simulink model "ACMtr_demo"  (R2019b)
settings: Solver=VariableStepAuto  StartTime=0.0  StopTime=2  RelTol=1e-3
libraries: powerlib x12, simulink x1
settings Model: Creator=DELL  LastModifiedBy=DELL

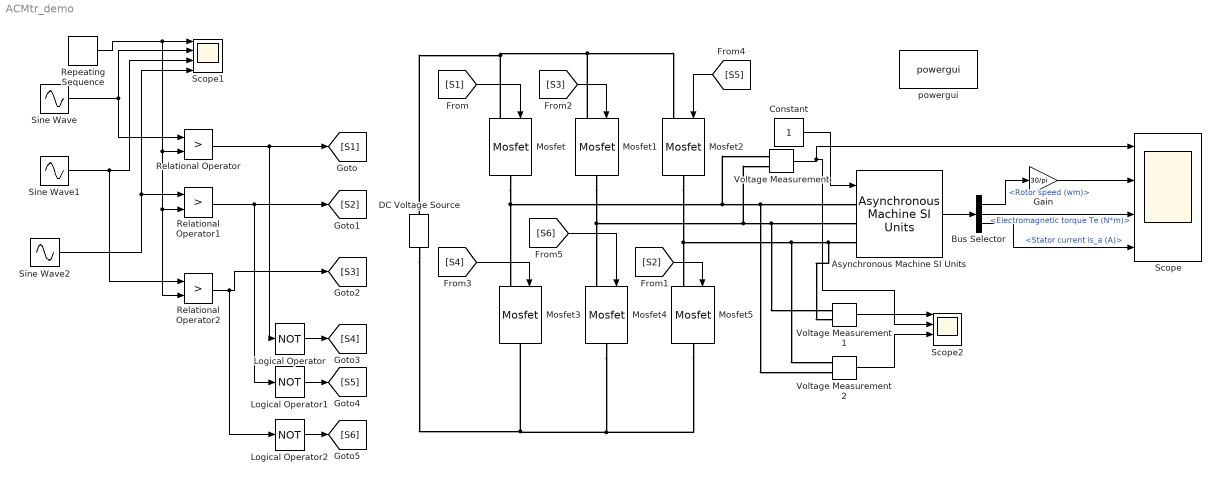
== system ACMtr_demo ==
  Asynchronous Machine SI Units : powerlib/Machines/Asynchronous Machine SI Units  RotorType=Squirrel-cage  PresetModel="15:  5.4 HP (4KW)   400 V  50Hz 1430 RPM"  MechanicalLoad=Torque Tm  ShowDetailedParameters=on  ReferenceFrame=Rotor  Units=SI  MeasurementBus=off  NominalParameters=[4000 400 50]  Stator=[1.405 0.005839]  Rotor=[1.395 0.005839]  Cage1=[0.4155 0.002066]  Cage2=[0.4168 0.0003495]  Lm=0.1722  Mechanical=[0.0131 0.002985 2]  PolePairs=2  InitialConditions=[0 0 0 0 0 0 0 0]  SimulateSaturation=off  Saturation=[14.03593122, 27.81365428, 53.79336849, 72.68890987, 97.98006896, 148.6815601, 215.7428561, 302.9841135, 428.7778367 ; 230, 322, 414, 460, 506, 552, 598, 644, 690]  LoadFlowParameters=1492000  TsPowergui=0  TsBlock=-1  IterativeModel=Trapezoidal non iterative  IterativeDiscreteModel=Trapezoidal non iterative  Pmec=1.492e+006
      settings: SourceProductName=Simscape Electrical
  Bus Selector : BusSelector  OutputSignals=Mechanical.Rotor speed (wm),Mechanical.Electromagnetic torque Te (N*m),Stator measurements.Stator current is_a (A)
  Constant : Constant
  DC Voltage Source : powerlib/Electrical Sources/DC Voltage Source  Amplitude=600  Measurements=None
      settings: SourceProductName=Simscape Electrical
  Gain : Gain  Gain=30/pi
  Logical Operator : Logic  Operator=NOT  AllPortsSameDT=off  OutDataTypeStr=boolean
  Logical Operator1 : Logic  Operator=NOT  AllPortsSameDT=off  OutDataTypeStr=boolean
  Logical Operator2 : Logic  Operator=NOT  AllPortsSameDT=off  OutDataTypeStr=boolean
  Mosfet{,1..5} (6 alike) : powerlib/Power Electronics/Mosfet  Ron=0.1  Lon=0  Rd=0.01  Vfd=0  IC=0  Rs=1e5  Cs=inf  Measurements=off
      settings: SourceProductName=Simscape Electrical
  Relational Operator : RelationalOperator  Operator=>  OutDataTypeStr=boolean  RndMeth=Simplest
  Relational Operator1 : RelationalOperator  Operator=>  OutDataTypeStr=boolean  RndMeth=Simplest
  Relational Operator2 : RelationalOperator  Operator=>  OutDataTypeStr=boolean  RndMeth=Simplest
  Repeating Sequence : simulink/Sources/Repeating Sequence  rep_seq_t=[0 0.25 0.5 0.75 1]/5000  rep_seq_y=[0 1 0 -1 0]
  Scope : Scope  NumInputPorts=4
  Scope1 : Scope  NumInputPorts=4
  Scope2 : Scope  NumInputPorts=4
  Sine Wave : Sin  Amplitude=0.6  Frequency=2*pi*50  SampleTime=0
  Sine Wave1 : Sin  Amplitude=0.6  Frequency=2*pi*50  Phase=120*pi/180  SampleTime=0
  Sine Wave2 : Sin  Amplitude=0.6  Frequency=2*pi*50  Phase=240*pi/180  SampleTime=0
  Voltage Measurement : powerlib/Measurements/Voltage Measurement  PhasorSimulation=off  OutputType=Complex  PSBequivalent=0
      settings: SourceProductName=Simscape Electrical
  Voltage Measurement1 : powerlib/Measurements/Voltage Measurement  PhasorSimulation=off  OutputType=Complex  PSBequivalent=0
      settings: SourceProductName=Simscape Electrical
  Voltage Measurement2 : powerlib/Measurements/Voltage Measurement  PhasorSimulation=off  OutputType=Complex  PSBequivalent=0
      settings: SourceProductName=Simscape Electrical
  powergui : powerlib/powergui  Priority=1  SimulationMode=Discrete  SampleTime=50e-6  frequency=60  Iterations=50  frequencyindice=50  Pbase=100e6  ErrMax=1e-4  UnitsV=kV  UnitsW=MW  buscounter=0  FunctionMessages=off  echomessages=off  EnableUseOfTLC=off  CurrentSourceSwitches=off  DisableSnubberDevices=off  DisableRonSwitches=off  DisableVfSwitches=off  DisplayEquations=off  AutomaticDiscreteSolvers=off  SolverType=Tustin/Backward Euler (TBE)  Interpol=off  ExternalGateDelay=off  methode=off  Ts=100  x0status=blocks  SPID=on  SwTol=0  HookPort=off  NonlinearTolerance=1e-4  nMaxIteration=100  ContinueOnMaxIteration=off  RestoreLinks=warning  ResistiveCurrentMeasurement=off  Frange=[0:2:500]  Ylog=off  Xlog=on  ShowGrid=off  save=off  variable=ZData  structure=0  ZoomFFT=off  StartTime=0.0  cycles=1  DisplayStyle=1  fundamental=60  FreqAxis=off  MaxFrequency=1000  frequencyindicesteady=1  RmsSteady=1  display=off
      settings: SourceProductName=Simscape Electrical
  wires:
  Relational Operator/1 -> Logical Operator/1, [S1]
  [S1] -> Mosfet/1
  [S2] -> Mosfet5/1
  Relational Operator2/1 -> Logical Operator2/1, [S3]
  [S3] -> Mosfet1/1
  Logical Operator/1 -> [S4]
  [S4] -> Mosfet3/1
  Logical Operator1/1 -> [S5]
  [S5] -> Mosfet2/1
  Logical Operator2/1 -> [S6]
  [S6] -> Mosfet4/1
  Constant/1 -> Asynchronous Machine SI Units/1
  Asynchronous Machine SI Units/1 -> Bus Selector/1
  Voltage Measurement/1 -> Scope2/2, Scope/1
  Bus Selector/1 -> Gain/1  "<Rotor speed (wm)>"
  Bus Selector/2 -> Scope/3  "<Electromagnetic torque Te (N*m)>"
  Bus Selector/3 -> Scope/4  "<Stator current is_a (A)>"
  Gain/1 -> Scope/2
  Repeating Sequence/1 -> Relational Operator2/2, Relational Operator1/2, Relational Operator/2, Scope1/1
  Sine Wave/1 -> Relational Operator/1, Scope1/2
  Sine Wave1/1 -> Relational Operator2/1, Scope1/3
  Sine Wave2/1 -> Relational Operator1/1, Scope1/4
  Relational Operator1/1 -> Logical Operator1/1, [S2]
  Voltage Measurement1/1 -> Scope2/1
  Voltage Measurement2/1 -> Scope2/3
  connections:
  Mosfet/RConn1 -- Voltage Measurement/LConn1 -- Voltage Measurement2/LConn2 -- Asynchronous Machine SI Units/LConn1 -- Mosfet3/LConn1
  Mosfet1/RConn1 -- Voltage Measurement/LConn2 -- Voltage Measurement1/LConn1 -- Asynchronous Machine SI Units/LConn2 -- Mosfet4/LConn1
  Mosfet2/RConn1 -- Voltage Measurement2/LConn1 -- Voltage Measurement1/LConn2 -- Asynchronous Machine SI Units/LConn3 -- Mosfet5/LConn1
  Mosfet5/RConn1 -- Mosfet4/RConn1 -- DC Voltage Source/LConn1 -- Mosfet3/RConn1
  Mosfet/LConn1 -- DC Voltage Source/RConn1 -- Mosfet1/LConn1 -- Mosfet2/LConn1
